simulink model "sampleModel1525_1"  (R2023a)
settings: Solver=VariableStepAuto  StartTime=0.0  StopTime=10.0  RelTol=1e-3
libraries: hdlsllib x5, simulink x1
settings Model: Creator=user1  LastModifiedBy=user1

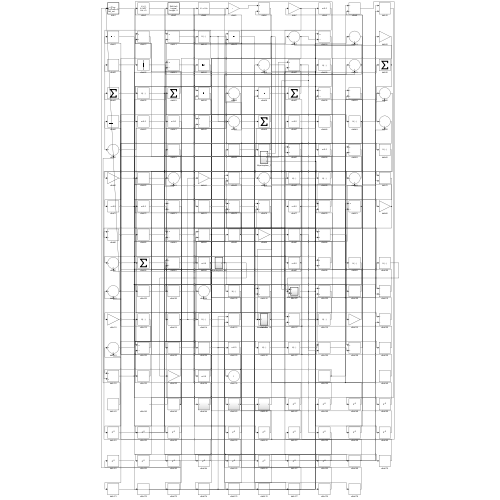
[thumbnail: Simulink's stored preview of the top-level diagram]
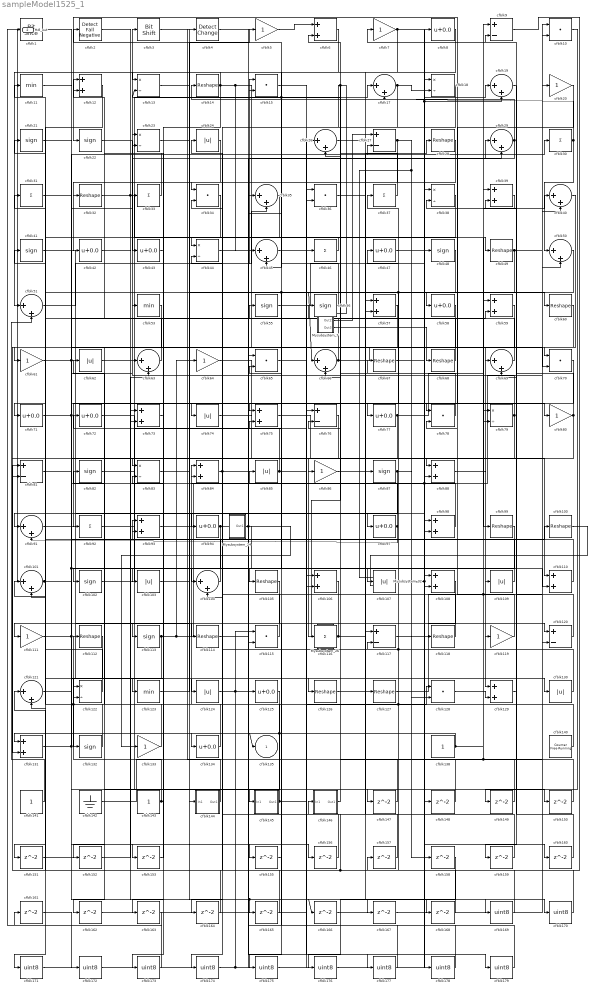
== system sampleModel1525_1 ==
  Mysubsystem_24 : Subsystem  TreatAsAtomicUnit=on  RTWFcnName=Mysubsystem_24
      settings: RTWFcnNameOpts=User specified  RTWFileNameOpts=Use function name
  Mysubsystem_26 : Subsystem  TreatAsAtomicUnit=on  RTWFcnName=Mysubsystem_26
      settings: RTWFcnNameOpts=User specified  RTWFileNameOpts=Use function name
  Mysubsystem_32 : Subsystem  TreatAsAtomicUnit=on  RTWFcnName=Mysubsystem_32
      settings: RTWFcnNameOpts=User specified  RTWFileNameOpts=Use function name
  Mysubsystem_7 : Subsystem  TreatAsAtomicUnit=on  RTWFcnName=Mysubsystem_7
      settings: RTWFcnNameOpts=User specified  RTWFileNameOpts=Use function name
  cfblk1 : hdlsllib/Logic and Bit Operations/Bit Slice  lidx=7  ridx=0
  cfblk{10,15,34,36,65,70,78,115,128} (9 alike) : DotProduct  OutDataTypeStr=uint8
  cfblk{14,28,32,49,60,67..68,99..100,105,112,114,118,126..127} (15 alike) : Reshape
  cfblk{17,19,26,29,35,40,45,50..51,63,66,69,91,101,104,121} (16 alike) : Sum  Inputs=|++  OutDataTypeStr=uint8
  cfblk{21..22,41,48,55..56,82,87,102,113,132} (11 alike) : Signum
  cfblk{24,62,74,85,103,107,109,124,130} (9 alike) : Abs  OutDataTypeStr=uint8  SaturateOnIntegerOverflow=off
  cfblk{6,12,39,57,59,73,75,84,88,93,98,106,108,110,129,131} (16 alike) : Sum  OutDataTypeStr=uint8
  cfblk11 : MinMax  OutDataTypeStr=uint8
  cfblk{5,7,20,61,64,80,86,111,119,133} (10 alike) : Gain  OutDataTypeStr=uint8
  cfblk{30..31,33,37,46,92,116} (7 alike) : Sum  Inputs=+  OutDataTypeStr=uint8
  cfblk{9,27,76,81,117,120} (6 alike) : Sum  Inputs=+-  OutDataTypeStr=uint8
  cfblk{13,18,23,38,44,79,83,122} (8 alike) : Product  Inputs=*/  OutDataTypeStr=uint8  RndMeth=Zero  SaturateOnIntegerOverflow=on
  cfblk123 : MinMax  OutDataTypeStr=uint8
  cfblk{8,42..43,47,58,71..72,77,94,97,125,134} (12 alike) : Bias  Bias=0.0  SaturateOnIntegerOverflow=off
  cfblk138 : Constant  OutDataTypeStr=uint8  SampleTime=-1
  cfblk140 : hdlsllib/Sources/Counter Free-Running  NumBits=16  tsamp=-1
  cfblk141 : Constant  OutDataTypeStr=uint8  SampleTime=-1
  cfblk142 : Ground
  cfblk143 : Constant  OutDataTypeStr=uint8  SampleTime=-1
  cfblk144 : Subsystem
      settings: LibrarySourceBlock=|
      | hdlsllib/Ports &
      | Subsystems/Subsystem
  cfblk145 : Subsystem
      settings: LibrarySourceBlock=|
      | hdlsllib/Ports &
      | Subsystems/Subsystem
  cfblk146 : Subsystem
      settings: LibrarySourceBlock=|
      | hdlsllib/Ports &
      | Subsystems/Subsystem
  cfblk{147..153,155..168} (21 alike) : Delay  SampleTime=1
  cfblk{169..179} (11 alike) : DataTypeConversion  OutDataTypeStr=uint8  SaturateOnIntegerOverflow=off  RndMeth=Floor
  cfblk2 : hdlsllib/Logic and Bit Operations/Detect Fall Negative  vinit=0  OutDataTypeStr=uint8
  cfblk3 : hdlsllib/Logic and Bit Operations/Bit Shift  mode=Shift Left Logical  N=0
  cfblk4 : simulink/Logic and Bit Operations/Detect Change  vinit=0  OutDataTypeStr=uint8
      settings: LibrarySourceBlock=|
      | hdlsllib/Logic and Bit
      | Operations/Detect
      | Change
  cfblk53 : MinMax  OutDataTypeStr=uint8
  cfblk135 : Outport  OutDataTypeStr=uint8  VectorParamsAs1DForOutWhenUnconnected=off
  Hdl_out : Outport  Port=2  OutDataTypeStr=uint8
  wires:
  cfblk44/1 -> cfblk58/1
  cfblk144/1(Out1) -> cfblk4/1
  cfblk61/1 -> cfblk97/1, cfblk56/1
  cfblk145/1(Out1) -> cfblk84/1, cfblk128/1
  cfblk119/1 -> cfblk22/1
  cfblk41/1 -> cfblk126/1
  cfblk5/1 -> cfblk6/1
  cfblk38/1 -> cfblk74/1
  cfblk102/1 -> cfblk17/1
  cfblk143/1 -> cfblk112/1, cfblk83/2
  cfblk112/1 -> cfblk132/1
  cfblk29/1 -> cfblk14/1, cfblk23/2
  cfblk6/1 -> cfblk51/1
  cfblk53/1 -> cfblk122/1
  cfblk46/1 -> cfblk44/1
  cfblk48/1 -> cfblk61/1
  cfblk72/1 -> cfblk130/1
  cfblk130/1 -> cfblk47/1, cfblk34/2
  cfblk125/1 -> cfblk135/1, cfblk162/1
  cfblk68/1 -> cfblk12/1
  cfblk88/1 -> cfblk129/1
  cfblk131/1 -> cfblk85/1, cfblk167/1
  cfblk80/1 -> cfblk7/1, cfblk94/1
  cfblk92/1 -> cfblk145/1(In1)
  cfblk116/1 -> cfblk111/1, cfblk28/1
  cfblk79/1 -> cfblk3/1, cfblk103/1
  cfblk3/1 -> cfblk60/1
  cfblk115/1 -> cfblk93/1
  cfblk40/1 -> cfblk70/1
  cfblk122/1 -> cfblk101/1
  cfblk28/1 -> cfblk42/1
  cfblk141/1 -> cfblk51/2
  cfblk64/1 -> cfblk110/1
  cfblk126/1 -> cfblk87/1
  cfblk47/1 -> cfblk8/1
  cfblk2/1 -> cfblk80/1
  cfblk91/1 -> cfblk144/1(In1)
  cfblk76/1 -> cfblk116/1
  cfblk98/1 -> cfblk37/1
  cfblk22/1 -> cfblk43/1
  cfblk30/1 -> cfblk50/1, cfblk17/2
  cfblk70/1 -> cfblk92/1
  cfblk59/1 -> cfblk119/1
  cfblk121/1 -> cfblk27/2
  cfblk66/1 -> cfblk69/1, cfblk55/1
  cfblk62/1 -> cfblk15/1
  cfblk86/1 -> cfblk30/1
  cfblk15/1 -> cfblk46/1
  cfblk93/1 -> cfblk59/1, cfblk48/1
  cfblk113/1 -> cfblk10/1, cfblk64/1, cfblk151/1
  cfblk107/1 -> cfblk19/1, cfblk19/2, cfblk160/1, cfblk158/1
  cfblk142/1 -> cfblk79/1, cfblk20/1
  cfblk138/1 -> cfblk9/1, cfblk131/1
  cfblk33/1 -> cfblk12/2
  cfblk69/1 -> cfblk24/1
  cfblk77/1 -> cfblk40/1, cfblk131/2
  cfblk99/1 -> cfblk102/1
  cfblk55/1 -> cfblk18/1
  cfblk56/1 -> cfblk2/1, cfblk13/2
  cfblk35/1 -> cfblk104/1
  cfblk104/1 -> cfblk72/1
  cfblk94/1 -> cfblk107/1, cfblk29/1, cfblk173/1
  cfblk8/1 -> cfblk57/2
  cfblk14/1 -> cfblk98/1, cfblk45/1, cfblk13/1, cfblk83/1
  cfblk87/1 -> cfblk118/1, cfblk171/1
  cfblk11/1 -> cfblk86/1
  cfblk1/1 -> cfblk75/1
  cfblk20/1 -> cfblk78/1
  cfblk36/1 -> cfblk169/1
  cfblk49/1 -> cfblk105/1, cfblk121/2, cfblk10/2
  cfblk83/1 -> cfblk59/2
  cfblk37/1 -> cfblk15/2
  cfblk26/1 -> cfblk49/1
  cfblk97/1 -> cfblk44/2, cfblk91/2
  cfblk117/1 -> cfblk120/1
  cfblk118/1 -> cfblk53/1
  cfblk45/1 -> cfblk88/1
  cfblk34/1 -> cfblk91/1
  cfblk39/1 -> cfblk38/2
  cfblk140/1 -> cfblk82/1, cfblk67/1
  cfblk50/1 -> cfblk66/1, cfblk77/1
  cfblk43/1 -> cfblk113/1
  cfblk32/1 -> cfblk165/1, cfblk166/1, cfblk99/1
  cfblk17/1 -> cfblk34/1, cfblk18/2
  cfblk133/1 -> cfblk122/2, cfblk41/1
  cfblk7/1 -> cfblk110/2, cfblk45/2
  cfblk74/1 -> cfblk127/1
  cfblk27/1 -> Mysubsystem_32/1(In1), cfblk128/2, cfblk32/1
  cfblk128/1 -> cfblk129/2
  cfblk111/1 -> cfblk100/1, cfblk153/1
  cfblk129/1 -> cfblk9/2
  cfblk71/1 -> cfblk124/1, cfblk106/2, cfblk33/1
  cfblk51/1 -> cfblk35/2
  cfblk127/1 -> cfblk79/2, cfblk40/2
  cfblk109/1 -> cfblk78/2
  cfblk108/1 -> cfblk174/1
  cfblk123/1 -> cfblk5/1
  cfblk120/1 -> cfblk39/2
  cfblk12/1 -> cfblk101/2
  cfblk24/1 -> cfblk73/2
  cfblk60/1 -> cfblk81/2
  cfblk85/1 -> cfblk62/1, cfblk98/2
  cfblk63/1 -> cfblk11/1
  cfblk57/1 -> cfblk71/1
  cfblk73/1 -> cfblk123/1
  cfblk82/1 -> cfblk26/1
  cfblk101/1 -> cfblk109/1, Hdl_out/1
  cfblk84/1 -> cfblk114/1, cfblk29/2
  cfblk134/1 -> cfblk23/1
  cfblk75/1 -> cfblk117/1
  cfblk23/1 -> cfblk88/2
  cfblk21/1 -> cfblk70/2
  cfblk110/1 -> cfblk31/1
  cfblk146/1(Out1) -> cfblk76/2
  cfblk132/1 -> cfblk21/1
  cfblk81/1 -> cfblk63/1
  cfblk78/1 -> cfblk26/2
  cfblk124/1 -> cfblk147/1
  cfblk147/1 -> cfblk6/2
  cfblk148/1 -> cfblk66/2
  cfblk10/1 -> cfblk149/1
  cfblk149/1 -> cfblk39/1
  cfblk31/1 -> cfblk150/1
  cfblk150/1 -> cfblk38/1
  cfblk151/1 -> cfblk63/2
  cfblk58/1 -> cfblk152/1
  cfblk152/1 -> cfblk73/1
  cfblk153/1 -> cfblk93/2
  cfblk42/1 -> cfblk155/1
  cfblk155/1 -> cfblk75/2
  cfblk13/1 -> cfblk156/1
  cfblk156/1 -> cfblk104/2
  cfblk9/1 -> cfblk157/1
  cfblk157/1 -> cfblk57/1
  cfblk19/1 -> cfblk159/1
  cfblk159/1 -> cfblk35/1
  cfblk160/1 -> cfblk69/2
  cfblk162/1 -> cfblk106/1
  cfblk105/1 -> cfblk163/1
  cfblk163/1 -> cfblk1/1
  cfblk18/1 -> cfblk164/1
  cfblk164/1 -> cfblk81/1
  cfblk165/1 -> cfblk121/1
  cfblk166/1 -> cfblk50/2
  cfblk167/1 -> cfblk120/2
  cfblk103/1 -> cfblk168/1
  cfblk168/1 -> cfblk117/2
  cfblk169/1 -> cfblk146/1(In1), cfblk84/2
  cfblk4/1 -> cfblk170/1
  cfblk170/1 -> cfblk36/1
  cfblk171/1 -> cfblk36/2
  cfblk161/1 -> cfblk172/1
  cfblk172/1 -> cfblk115/2
  cfblk173/1 -> cfblk161/1
  cfblk174/1 -> cfblk125/1, cfblk115/1, cfblk148/1
  cfblk106/1 -> cfblk175/1
  cfblk175/1 -> cfblk108/1
  cfblk158/1 -> cfblk176/1
  cfblk176/1 -> cfblk108/2
  cfblk65/1 -> cfblk177/1
  cfblk177/1 -> cfblk76/1
  cfblk67/1 -> cfblk178/1
  cfblk178/1 -> cfblk65/1
  cfblk114/1 -> cfblk179/1
  cfblk179/1 -> cfblk65/2
  Mysubsystem_7/1(Out1) -> Mysubsystem_26/1(In1), cfblk134/1
  Mysubsystem_7/2(Out2) -> cfblk27/1
  Mysubsystem_7/3(Out3) -> cfblk68/1
  Mysubsystem_24/1(Out1) -> cfblk133/1
  cfblk100/1 -> Mysubsystem_32/2(In2)

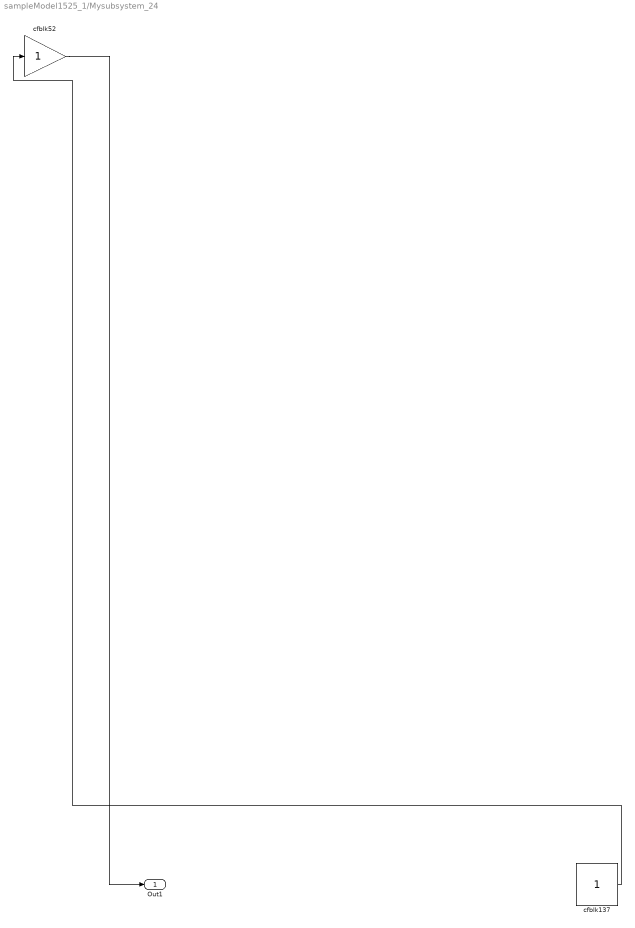
== system sampleModel1525_1/Mysubsystem_24 ==
  cfblk137 : Constant  SampleTime=-1
  cfblk52 : Gain
  Out1 : Outport
  wires:
  cfblk137/1 -> cfblk52/1
  cfblk52/1 -> Out1/1

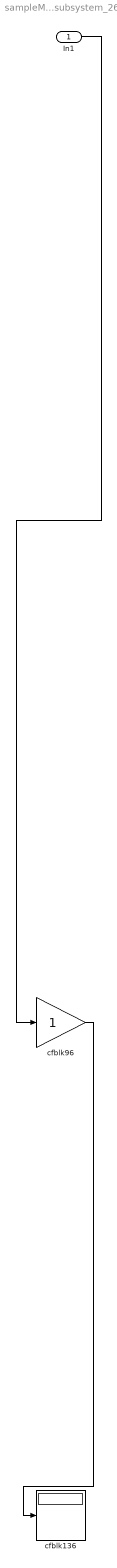
== system sampleModel1525_1/Mysubsystem_26 ==
  In1 : Inport
  cfblk136 : Display
  cfblk96 : Gain
  wires:
  In1/1 -> cfblk96/1
  cfblk96/1 -> cfblk136/1

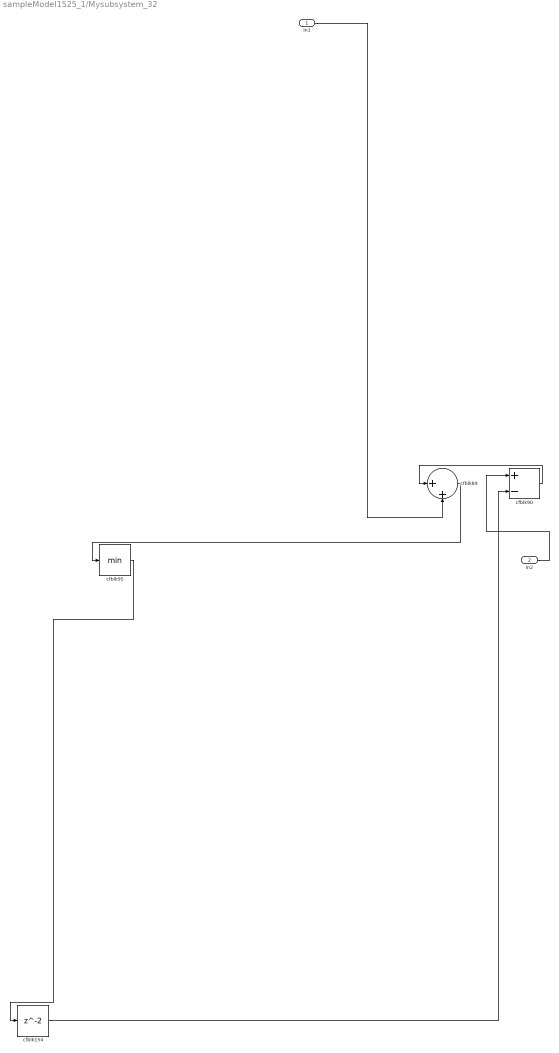
== system sampleModel1525_1/Mysubsystem_32 ==
  In1 : Inport
  In2 : Inport  Port=2
  cfblk154 : Delay  SampleTime=1
  cfblk89 : Sum  Inputs=|++
  cfblk90 : Sum  Inputs=+-
  cfblk95 : MinMax
  wires:
  cfblk90/1 -> cfblk89/1
  cfblk154/1 -> cfblk90/2
  In1/1 -> cfblk89/2
  cfblk89/1 -> cfblk95/1
  cfblk95/1 -> cfblk154/1
  In2/1 -> cfblk90/1

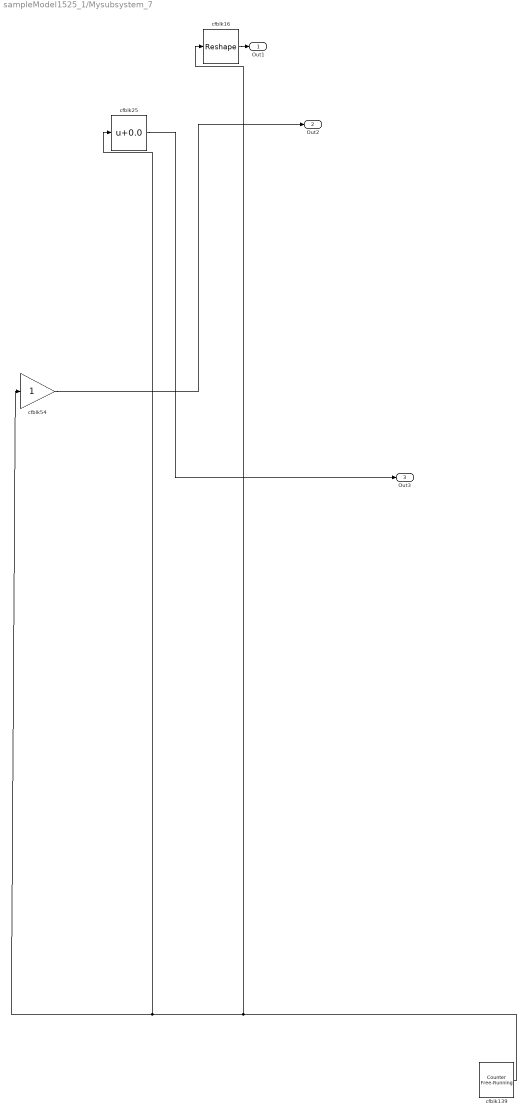
== system sampleModel1525_1/Mysubsystem_7 ==
  cfblk139 : hdlsllib/Sources/Counter Free-Running  NumBits=16  tsamp=-1
  cfblk16 : Reshape
  cfblk25 : Bias  Bias=0.0  SaturateOnIntegerOverflow=off
  cfblk54 : Gain
  Out1 : Outport
  Out2 : Outport  Port=2
  Out3 : Outport  Port=3
  wires:
  cfblk139/1 -> cfblk54/1, cfblk25/1, cfblk16/1
  cfblk16/1 -> Out1/1
  cfblk54/1 -> Out2/1
  cfblk25/1 -> Out3/1

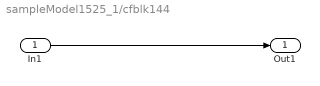
== system sampleModel1525_1/cfblk144 ==
  In1 : Inport
  Out1 : Outport
  wires:
  In1/1 -> Out1/1

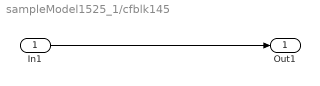
== system sampleModel1525_1/cfblk145 ==
  In1 : Inport
  Out1 : Outport
  wires:
  In1/1 -> Out1/1

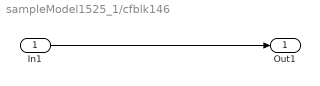
== system sampleModel1525_1/cfblk146 ==
  In1 : Inport
  Out1 : Outport
  wires:
  In1/1 -> Out1/1
